simulink model "fftanalyzeri"  (R2012b)
settings: Solver=ode3  SolverMode=SingleTasking  StartTime=0.0  StopTime=20000  RelTol=1e-3
undefined symbols (not defined in the file or in its folder): pfb_coeff_gen_calc
undefined symbols (not defined in the file): fft_bin_flags_, magphmeanmem_, threshmem_
libraries: xbsIndex_r4 x9073, casper_library_misc x119, casper_library_flow_control x51, casper_library_delays x22, xps_library x10
(part 2 of 74)

== system fftanalyzeri/BinData ==
  addr : Inport
  data_in : Inport  Port=2
  we : Inport  Port=3
  calc_add : Subsystem  mask{data_width=32, addr_width=10, sample_rate=sample_rate}
      mask prompts: data_width "data width"; addr_width "address width"; sample_rate "sample rate"
  convert_addr : xbsIndex_r4/Convert  gui_display_data_type=Fixed-point  arith_type=Unsigned  n_bits=addr_width  bin_pt=0  float_type=Single  exp_bits=8  fraction_bits=24  quantization=Truncate  overflow=Wrap  en=off  latency=0  dbl_ovrd=off  pipeline=off  block_type=convert
      settings: xl_area=[0, 0, 0, 0, 0, 0, 0]
  convert_din1 : xbsIndex_r4/Convert  gui_display_data_type=Fixed-point  arith_type=Unsigned  n_bits=32  bin_pt=0  float_type=Single  exp_bits=8  fraction_bits=24  quantization=Truncate  overflow=Wrap  en=off  latency=0  dbl_ovrd=off  pipeline=off  block_type=convert
      settings: xl_area=[0, 0, 0, 0, 0, 0, 0]
  convert_we : xbsIndex_r4/Convert  gui_display_data_type=Fixed-point  arith_type=Unsigned  n_bits=1  bin_pt=0  float_type=Single  exp_bits=8  fraction_bits=24  quantization=Truncate  overflow=Wrap  en=off  latency=0  dbl_ovrd=off  pipeline=off  block_type=convert
      settings: xl_area=[0, 0, 0, 0, 0, 0, 0]
  fftanalyzeri_BinData_addr : xbsIndex_r4/Gateway Out  inherit_from_input=off  hdl_port=on  timing_constraint=None  locs_specified=off  LOCs={'A5','B9','A9','C1','A3','G6','E9','A6','A7','A8','B8','B1','B3','D9','B5','B4','B6','C2'}  UseAsDAC=off  DACChannel='1'  block_type=gatewayout
      settings: infoedit="Gateway out block.  Converts Xilinx fixed point inputs into ouputs of type Simulink integer, double, or fixed point.<P><P>Hardware notes:  In hardware these blocks become top level output ports or are discarded, depending on how they are configured."  xl_area=[0, 0, 0, 0, 0, 0, 0]  sginterface={'Nallatech'=>{'xdspkit'=>{'non_memory_mapped_port'=>'uprev_Shared_BRAM_addr'}},'Xilinx'=>{'jtaghwcosim'=>{'non_memory_mapped_port'=>'uprev_Shared_BRAM_addr'},'xdspkit'=>{'non_memory_mapped_port'=>'uprev_Shared_BRAM_addr'}}}
  fftanalyzeri_BinData_data_in : xbsIndex_r4/Gateway Out  inherit_from_input=off  hdl_port=on  timing_constraint=None  locs_specified=off  LOCs={'B21','B22','A22','B23','B19','C19','A20','A21','A23','B24','A24','A25','E18','D18','C18','B18'}  UseAsDAC=off  DACChannel='1'  block_type=gatewayout
      settings: infoedit="Gateway out block.  Converts Xilinx fixed point inputs into ouputs of type Simulink integer, double, or fixed point.<P><P>Hardware notes:  In hardware these blocks become top level output ports or are discarded, depending on how they are configured."  xl_area=[0, 0, 0, 0, 0, 0, 0]  sginterface={'Nallatech'=>{'xdspkit'=>{'non_memory_mapped_port'=>'uprev_Shared_BRAM_data_in'}},'Xilinx'=>{'jtaghwcosim'=>{'non_memory_mapped_port'=>'uprev_Shared_BRAM_data_in'},'xdspkit'=>{'non_memory_mapped_port'=>'uprev_Shared_BRAM_data_in'}}}
  fftanalyzeri_BinData_data_out : xbsIndex_r4/Gateway In  gui_display_data_type=Fixed-point  arith_type=Unsigned  n_bits=32  bin_pt=0  preci_type=Single  exp_width=8  frac_width=24  quantization=Truncate  overflow=Wrap  period=sample_rate  dbl_ovrd=off  timing_constraint=None  locs_specified=off  LOCs={}  UseAsADC=off  ADCChannel='1'  inherit_from_input=off  hdl_port=on  block_type=gatewayin
      settings: xl_area=[0, 0, 0, 0, 0, 0, 0]
  fftanalyzeri_BinData_we : xbsIndex_r4/Gateway Out  inherit_from_input=off  hdl_port=on  timing_constraint=None  locs_specified=off  LOCs={'A14'}  UseAsDAC=off  DACChannel='1'  block_type=gatewayout
      settings: infoedit="Gateway out block.  Converts Xilinx fixed point inputs into ouputs of type Simulink integer, double, or fixed point.<P><P>Hardware notes:  In hardware these blocks become top level output ports or are discarded, depending on how they are configured."  xl_area=[0, 0, 0, 0, 0, 0, 0]
  mem : Subsystem
  munge_in : Subsystem  AncestorBlock=casper_library_flow_control/munge  mask(munge){divisions=1, div_size=32, order=[0], arith_type_out=Unsigned, bin_pt_out=0}
      mask prompts: divisions "Number of divisions"; div_size "Division size (bits)"; order "Division packing order"; arith_type_out "Output arithmetic type"; bin_pt_out "Output binary point"
      mask help: Splits an input bus into the specified number of divisions and then recombines them in the order specified (most significant division = 0,least = number divisions-1)
      mask init:
      | munge_init(gcb, ...
      |     'divisions', divisions, ...
      |     'div_size', div_size, ...
      |     'order', order, ...
      |     'arith_type_out', arith_type_out, ...
      |     'bin_pt_out', bin_pt_out);
      settings: AttributesFormatString=|
      | split:32
      | join:0
      | Unsigned [32,0]
      mask TypeOptions arith_type_out: Unsigned | Signed  (2's comp) | Floating-point
  munge_out : Subsystem  AncestorBlock=casper_library_flow_control/munge  mask(munge){divisions=1, div_size=32, order=[0], arith_type_out=Unsigned, bin_pt_out=0}
      mask prompts: divisions "Number of divisions"; div_size "Division size (bits)"; order "Division packing order"; arith_type_out "Output arithmetic type"; bin_pt_out "Output binary point"
      mask help: Splits an input bus into the specified number of divisions and then recombines them in the order specified (most significant division = 0,least = number divisions-1)
      mask init:
      | munge_init(gcb, ...
      |     'divisions', divisions, ...
      |     'div_size', div_size, ...
      |     'order', order, ...
      |     'arith_type_out', arith_type_out, ...
      |     'bin_pt_out', bin_pt_out);
      settings: AttributesFormatString=|
      | split:32
      | join:0
      | Unsigned [32,0]
      mask TypeOptions arith_type_out: Unsigned | Signed  (2's comp) | Floating-point
  data_out : Outport
  wires:
  convert_addr/1 -> fftanalyzeri_BinData_addr/1
  convert_din1/1 -> fftanalyzeri_BinData_data_in/1
  data_in/1 -> munge_in/1(din)
  calc_add/1(out) -> convert_addr/1
  fftanalyzeri_BinData_we/1 -> mem/3(In3)
  fftanalyzeri_BinData_data_in/1 -> mem/2(In2)
  fftanalyzeri_BinData_addr/1 -> mem/1(In1)
  convert_we/1 -> fftanalyzeri_BinData_we/1
  fftanalyzeri_BinData_data_out/1 -> munge_out/1(din)
  mem/1(Out1) -> fftanalyzeri_BinData_data_out/1
  addr/1 -> calc_add/1(in)
  we/1 -> convert_we/1
  munge_out/1(dout) -> data_out/1
  munge_in/1(dout) -> convert_din1/1

== system fftanalyzeri/DRAM_LUT ==
  LUTsize : Inport
  startDAC : Inport  Port=2
  sys_sync : Inport  Port=3
  resetDRAM : Inport  Port=4
  RWen : Inport  Port=5
  holdcounter : Inport  Port=6
  seeaddress : Inport  Port=7
  Constant : xbsIndex_r4/Constant  const=0  gui_display_data_type=Fixed-point  arith_type=Unsigned  n_bits=32  bin_pt=0  preci_type=Single  exp_width=8  frac_width=24  explicit_period=off  period=1  equ=P=C  opselect=C  inp2=PCIN>>17  opr=+  inp1=P  carry=CIN  dbl_ovrd=off  block_type=constant
      settings: block_version=11.4
  Constant2 : xbsIndex_r4/Constant  const=0  gui_display_data_type=Fixed-point  arith_type=Unsigned  n_bits=144  bin_pt=0  preci_type=Single  exp_width=8  frac_width=24  explicit_period=on  period=1  equ=P=C  opselect=C  inp2=PCIN>>17  opr=+  inp1=P  carry=CIN  dbl_ovrd=off  block_type=constant
  Constant3 : xbsIndex_r4/Constant  const=0  gui_display_data_type=Fixed-point  arith_type=Unsigned  n_bits=36  bin_pt=0  preci_type=Single  exp_width=8  frac_width=24  explicit_period=on  period=1  equ=P=C  opselect=C  inp2=PCIN>>17  opr=+  inp1=P  carry=CIN  dbl_ovrd=off  block_type=constant
  Constant4 : xbsIndex_r4/Constant  const=0  gui_display_data_type=Fixed-point  arith_type=Unsigned  n_bits=32  bin_pt=0  preci_type=Single  exp_width=8  frac_width=24  explicit_period=on  period=1  equ=P=C  opselect=C  inp2=PCIN>>17  opr=+  inp1=P  carry=CIN  dbl_ovrd=off  block_type=constant
  Convert3 : xbsIndex_r4/Convert  gui_display_data_type=Fixed-point  arith_type=Unsigned  n_bits=32  bin_pt=0  float_type=Single  exp_bits=8  fraction_bits=24  quantization=Truncate  overflow=Wrap  en=off  latency=0  dbl_ovrd=off  pipeline=off  block_type=convert
      settings: block_version=10.1.3
  Counter1 : xbsIndex_r4/Counter  cnt_type=Free Running  cnt_to=511  operation=Up  start_count=0  cnt_by_val=1  arith_type=Unsigned  n_bits=32  bin_pt=0  load_pin=off  rst=on  en=on  explicit_period=on  period=1  dbl_ovrd=off  use_behavioral_HDL=off  implementation=Fabric  use_rpm=off  block_type=counter
  Counter2 : xbsIndex_r4/Counter  cnt_type=Free Running  cnt_to=512  operation=Up  start_count=0  cnt_by_val=1  arith_type=Unsigned  n_bits=32  bin_pt=0  load_pin=off  rst=on  en=on  explicit_period=on  period=1  dbl_ovrd=off  use_behavioral_HDL=off  implementation=Fabric  use_rpm=off  block_type=counter
  Delay4 : xbsIndex_r4/Delay  rst=off  infoeditControl=Selection of Reset will increase slice count due to use of real FFs and instead of SRLs  en=off  latency=2  dbl_ovrd=off  reg_retiming=off  block_type=delay
  Gateway Out{,1..7} (8 alike) : xbsIndex_r4/Gateway Out  inherit_from_input=off  hdl_port=on  timing_constraint=None  locs_specified=off  LOCs={}  UseAsDAC=off  DACChannel='1'  block_type=gatewayout
  Inverter1 : xbsIndex_r4/Inverter  en=off  latency=0  dbl_ovrd=off  block_type=inv
  Logical2 : xbsIndex_r4/Logical  logical_function=OR  inputs=2  en=off  latency=0  precision=Full  arith_type=Unsigned  n_bits=16  bin_pt=0  align_bp=on  dbl_ovrd=off  block_type=logical
  Mux : xbsIndex_r4/Mux  inputs=2  en=off  latency=0  precision=Full  arith_type=Unsigned  n_bits=16  bin_pt=14  quantization=Truncate  overflow=Wrap  dbl_ovrd=off  block_type=mux
      settings: block_version=11.4
  Mux1 : xbsIndex_r4/Mux  inputs=2  en=off  latency=0  precision=Full  arith_type=Unsigned  n_bits=16  bin_pt=14  quantization=Truncate  overflow=Wrap  dbl_ovrd=off  block_type=mux
  Reinterpret{1..8} (8 alike) : xbsIndex_r4/Reinterpret  force_arith_type=on  arith_type="Signed  (2's comp)"  force_bin_pt=on  bin_pt=15  block_type=reinterpret
      settings: infoedit="Changes signal type without altering the binary representation.   You can changed the signal between signed and unsigned, and relocate the binary point.<P><P>Hardware notes: In hardware this block costs nothing.<P><P>Example:  Suppose the input is 6 bits wide, signed, with 2 fractional bits, and the output is forced to unsigned with 0 fractional bits.  Then an input of -2.0 (1110.00 in binary 2's complement) becomes an output of 56 (111000 in binary)."  block_version=10.1.3
  Relational2 : xbsIndex_r4/Relational  mode=a=b  en=off  latency=0  dbl_ovrd=off  block_type=relational
      settings: block_version=10.1.3
  Slice10 : xbsIndex_r4/Slice  nbits=1  boolean_output=on  mode=Lower Bit Location + Width  bit1=0  base1=MSB of Input  bit0=0  base0=LSB of Input  dbl_ovrd=off  block_type=slice
      settings: infoedit="Extracts a given range of bits from each input sample and presents it at the output.  The output type is ordinarily unsigned with binary point at zero, but can be Boolean when the slice is one bit wide.<P><P>Hardware notes: In hardware this block costs nothing."  block_version=10.1.3
  Slice_16_0_ : xbsIndex_r4/Slice  nbits=16  boolean_output=off  mode=Lower Bit Location + Width  bit1=0  base1=LSB of Input  bit0=0  base0=LSB of Input  dbl_ovrd=off  block_type=slice
  Slice_16_0_1 : xbsIndex_r4/Slice  nbits=16  boolean_output=off  mode=Lower Bit Location + Width  bit1=0  base1=LSB of Input  bit0=0  base0=LSB of Input  dbl_ovrd=off  block_type=slice
  Slice_16_104_6 : xbsIndex_r4/Slice  nbits=16  boolean_output=off  mode=Lower Bit Location + Width  bit1=0  base1=LSB of Input  bit0=104  base0=LSB of Input  dbl_ovrd=off  block_type=slice
  Slice_16_120_7 : xbsIndex_r4/Slice  nbits=16  boolean_output=off  mode=Lower Bit Location + Width  bit1=0  base1=LSB of Input  bit0=120  base0=LSB of Input  dbl_ovrd=off  block_type=slice
  Slice_16_16_1 : xbsIndex_r4/Slice  nbits=16  boolean_output=off  mode=Lower Bit Location + Width  bit1=0  base1=LSB of Input  bit0=16  base0=LSB of Input  dbl_ovrd=off  block_type=slice
  Slice_16_32_2 : xbsIndex_r4/Slice  nbits=16  boolean_output=off  mode=Lower Bit Location + Width  bit1=0  base1=LSB of Input  bit0=32  base0=LSB of Input  dbl_ovrd=off  block_type=slice
  Slice_16_64_3 : xbsIndex_r4/Slice  nbits=16  boolean_output=off  mode=Lower Bit Location + Width  bit1=0  base1=LSB of Input  bit0=48  base0=LSB of Input  dbl_ovrd=off  block_type=slice
  Slice_16_72_4 : xbsIndex_r4/Slice  nbits=16  boolean_output=off  mode=Lower Bit Location + Width  bit1=0  base1=LSB of Input  bit0=72  base0=LSB of Input  dbl_ovrd=off  block_type=slice
  Slice_16_88_5 : xbsIndex_r4/Slice  nbits=16  boolean_output=off  mode=Lower Bit Location + Width  bit1=0  base1=LSB of Input  bit0=88  base0=LSB of Input  dbl_ovrd=off  block_type=slice
  dram : xps_library/dram  Tag=xps:dram  dimm=1  arith_type=Unsigned  bin_pt=0  ip_clock=200  sample_period=1  bram_fifos=on  disable_tag=off  ram_depth=18  bank_mgt=off  wide_data=off  half_burst=off  use_sniffer=on
  memscope : Scope  NumInputPorts=8
      settings: YMin=-5~-5~-5~-5~-5~-5~-5~-5  YMax=5~5~5~5~5~5~5~5
  posedge : casper_library_misc/posedge  Tag=Rising Edge Detector
  posedge2 : casper_library_misc/posedge  Tag=Rising Edge Detector
  data_i0 : Outport
  data_i1 : Outport  Port=2
  data_i2 : Outport  Port=3
  data_i3 : Outport  Port=4
  data_q0 : Outport  Port=5
  data_q1 : Outport  Port=6
  data_q2 : Outport  Port=7
  data_q3 : Outport  Port=8
  sync_out : Outport  Port=9
  wires:
  resetDRAM/1 -> dram/1, Gateway Out/1
  RWen/1 -> Gateway Out2/1, dram/5, dram/8
  Constant2/1 -> dram/3
  Constant3/1 -> dram/4
  Counter2/1 -> Relational2/2, Gateway Out4/1, Mux/2
  Counter1/1 -> Slice10/1
  Slice10/1 -> posedge2/1
  Convert3/1 -> Relational2/1
  posedge2/1 -> Counter2/2, Delay4/1
  Constant4/1 -> dram/6
  Delay4/1 -> Gateway Out3/1, dram/7
  LUTsize/1 -> Convert3/1
  Slice_16_16_1/1 -> Reinterpret1/1
  Slice_16_104_6/1 -> Reinterpret3/1
  Slice_16_120_7/1 -> Reinterpret2/1
  Slice_16_32_2/1 -> Reinterpret5/1
  Slice_16_64_3/1 -> Reinterpret6/1
  Slice_16_88_5/1 -> Reinterpret7/1
  Slice_16_72_4/1 -> Reinterpret8/1
  Reinterpret4/1 -> data_i0/1
  Reinterpret1/1 -> data_i1/1
  Reinterpret5/1 -> data_i2/1
  Reinterpret6/1 -> data_i3/1
  Reinterpret8/1 -> data_q0/1
  Reinterpret7/1 -> data_q1/1
  Reinterpret3/1 -> data_q2/1
  Reinterpret2/1 -> data_q3/1
  startDAC/1 -> Inverter1/1, Counter1/2
  Logical2/1 -> Counter2/1
  Relational2/1 -> posedge/1, Logical2/1
  Inverter1/1 -> Logical2/2
  sys_sync/1 -> Counter1/1
  Mux/1 -> dram/2, Slice_16_0_1/1, Gateway Out1/1
  Constant/1 -> Mux/3
  holdcounter/1 -> Mux/1
  Gateway Out/1 -> memscope/1
  Gateway Out1/1 -> memscope/2
  Gateway Out2/1 -> memscope/3
  Gateway Out3/1 -> memscope/4
  Gateway Out4/1 -> memscope/5
  Gateway Out5/1 -> memscope/6
  dram/2 -> Slice_16_120_7/1, Slice_16_104_6/1, Slice_16_88_5/1, Slice_16_72_4/1, Slice_16_64_3/1, Slice_16_32_2/1, Slice_16_16_1/1, Slice_16_0_/1, Gateway Out7/1
  Gateway Out7/1 -> memscope/7
  Gateway Out6/1 -> memscope/8
  dram/4 -> Gateway Out6/1
  dram/1 -> Gateway Out5/1
  Slice_16_0_/1 -> Mux1/2
  Mux1/1 -> Reinterpret4/1
  Slice_16_0_1/1 -> Mux1/3
  seeaddress/1 -> Mux1/1
  posedge/1 -> sync_out/1

== system fftanalyzeri/FIFO64_ ==
  chanwr : Inport
  wr : Inport  Port=2
  din : Inport  Port=3
  chanrd : Inport  Port=4
  rd : Inport  Port=5
  rst : Inport  Port=6
  rden : Inport  Port=7
  wren : Inport  Port=8
  FIFO32_0 : Subsystem
  FIFO32_1 : Subsystem
  Gateway Out{1..16} (16 alike) : xbsIndex_r4/Gateway Out  inherit_from_input=off  hdl_port=on  timing_constraint=None  locs_specified=off  LOCs={}  UseAsDAC=off  DACChannel='1'  block_type=gatewayout
  Subsystem1 : Subsystem
  Subsystem2 : Subsystem
  fifoscope1 : Scope  NumInputPorts=8
      settings: YMin=-5~-5~-5~-5~-5~-5~-5~-5  YMax=5~5~5~5~5~5~5~5  SaveName=fsmdata6
  fifoscope2 : Scope  NumInputPorts=8
      settings: YMin=-5~-5~-5~-5~-5~-5~-5~-5  YMax=5~5~5~5~5~5~5~5  SaveName=fsmdata7
  q : Outport
  empty : Outport  Port=2
  halffull : Outport  Port=3
  quartfull : Outport  Port=4
  threeqfull : Outport  Port=5
  full : Outport  Port=6
  fifllen : Outport  Port=7
  dvld : Outport  Port=8
  wires:
  wr/1 -> Gateway Out10/1, FIFO32_1/2(wr), FIFO32_0/2(wr)
  rst/1 -> FIFO32_1/6(rst), FIFO32_0/6(rst)
  chanrd/1 -> Gateway Out9/1, Subsystem2/2(chanrd), Subsystem1/4(In4), FIFO32_1/4(chanrd), FIFO32_0/4(chanrd)
  din/1 -> FIFO32_1/3(din), FIFO32_0/3(din)
  chanwr/1 -> Gateway Out8/1, Subsystem2/1(chanwr), FIFO32_1/1(chanwr), FIFO32_0/1(chanwr)
  rd/1 -> Gateway Out11/1, FIFO32_1/5(rd), FIFO32_0/5(rd)
  FIFO32_0/1(q) -> Subsystem1/1(In1)
  FIFO32_0/2(empty) -> Gateway Out7/1, Subsystem1/2(In2)
  FIFO32_0/3(halffull) -> Gateway Out1/1, Subsystem1/3(In3)
  FIFO32_0/4(quartfull) -> Gateway Out2/1, Subsystem1/5(In5)
  FIFO32_0/5(threeqfull) -> Subsystem1/6(In6)
  FIFO32_0/6(full) -> Subsystem1/7(In7)
  FIFO32_0/7(fifllen) -> Gateway Out16/1, Subsystem1/8(In8)
  FIFO32_0/8(dvld) -> Subsystem1/9(In9)
  FIFO32_1/1(q) -> Subsystem1/10(In10)
  FIFO32_1/2(empty) -> Gateway Out3/1, Subsystem1/11(In11)
  FIFO32_1/3(halffull) -> Subsystem1/12(In12)
  FIFO32_1/4(quartfull) -> Gateway Out5/1, Subsystem1/13(In13)
  FIFO32_1/5(threeqfull) -> Gateway Out6/1, Subsystem1/14(In14)
  FIFO32_1/6(full) -> Subsystem1/15(In15)
  FIFO32_1/7(fifllen) -> Gateway Out4/1, Subsystem1/16(In16)
  FIFO32_1/8(dvld) -> Subsystem1/17(In17)
  Subsystem1/1(Out1) -> q/1
  Subsystem1/2(Out2) -> empty/1
  Subsystem1/3(Out3) -> halffull/1
  Subsystem1/4(Out4) -> quartfull/1
  Subsystem1/5(Out5) -> threeqfull/1
  Subsystem1/6(Out6) -> full/1
  Subsystem1/7(Out7) -> fifllen/1
  Subsystem1/8(Out8) -> dvld/1
  rden/1 -> Subsystem2/3(rden)
  wren/1 -> Subsystem2/4(wren)
  Subsystem2/2(rdl) -> Gateway Out13/1, FIFO32_0/7(rden)
  Subsystem2/3(wrh) -> Gateway Out14/1, FIFO32_1/8(wren)
  Subsystem2/1(wrl) -> Gateway Out12/1, FIFO32_0/8(wren)
  Subsystem2/4(rdh) -> Gateway Out15/1, FIFO32_1/7(rden)
  Gateway Out8/1 -> fifoscope1/1
  Gateway Out9/1 -> fifoscope1/2
  Gateway Out10/1 -> fifoscope1/3
  Gateway Out11/1 -> fifoscope1/4
  Gateway Out12/1 -> fifoscope1/5
  Gateway Out13/1 -> fifoscope1/6
  Gateway Out14/1 -> fifoscope1/7
  Gateway Out15/1 -> fifoscope1/8
  Gateway Out7/1 -> fifoscope2/1
  Gateway Out16/1 -> fifoscope2/2
  Gateway Out1/1 -> fifoscope2/3
  Gateway Out2/1 -> fifoscope2/4
  Gateway Out3/1 -> fifoscope2/5
  Gateway Out4/1 -> fifoscope2/6
  Gateway Out5/1 -> fifoscope2/7
  Gateway Out6/1 -> fifoscope2/8

== system fftanalyzeri/FIFO64_1 ==
  chanwr : Inport
  wr : Inport  Port=2
  din : Inport  Port=3
  chanrd : Inport  Port=4
  rd : Inport  Port=5
  rst : Inport  Port=6
  rden : Inport  Port=7
  wren : Inport  Port=8
  FIFO32_0 : Subsystem
  FIFO32_1 : Subsystem
  Subsystem1 : Subsystem
  Subsystem2 : Subsystem
  q : Outport
  empty : Outport  Port=2
  halffull : Outport  Port=3
  quartfull : Outport  Port=4
  threeqfull : Outport  Port=5
  full : Outport  Port=6
  fifllen : Outport  Port=7
  dvld : Outport  Port=8
  wires:
  wr/1 -> FIFO32_1/2(wr), FIFO32_0/2(wr)
  rst/1 -> FIFO32_1/6(rst), FIFO32_0/6(rst)
  chanrd/1 -> Subsystem2/2(chanrd), Subsystem1/4(In4), FIFO32_1/4(chanrd), FIFO32_0/4(chanrd)
  din/1 -> FIFO32_1/3(din), FIFO32_0/3(din)
  chanwr/1 -> Subsystem2/1(chanwr), FIFO32_1/1(chanwr), FIFO32_0/1(chanwr)
  rd/1 -> FIFO32_1/5(rd), FIFO32_0/5(rd)
  FIFO32_0/1(q) -> Subsystem1/1(In1)
  FIFO32_0/2(empty) -> Subsystem1/2(In2)
  FIFO32_0/3(halffull) -> Subsystem1/3(In3)
  FIFO32_0/4(quartfull) -> Subsystem1/5(In5)
  FIFO32_0/5(threeqfull) -> Subsystem1/6(In6)
  FIFO32_0/6(full) -> Subsystem1/7(In7)
  FIFO32_0/7(fifllen) -> Subsystem1/8(In8)
  FIFO32_0/8(dvld) -> Subsystem1/9(In9)
  FIFO32_1/1(q) -> Subsystem1/10(In10)
  FIFO32_1/2(empty) -> Subsystem1/11(In11)
  FIFO32_1/3(halffull) -> Subsystem1/12(In12)
  FIFO32_1/4(quartfull) -> Subsystem1/13(In13)
  FIFO32_1/5(threeqfull) -> Subsystem1/14(In14)
  FIFO32_1/6(full) -> Subsystem1/15(In15)
  FIFO32_1/7(fifllen) -> Subsystem1/16(In16)
  FIFO32_1/8(dvld) -> Subsystem1/17(In17)
  Subsystem1/1(Out1) -> q/1
  Subsystem1/2(Out2) -> empty/1
  Subsystem1/3(Out3) -> halffull/1
  Subsystem1/4(Out4) -> quartfull/1
  Subsystem1/5(Out5) -> threeqfull/1
  Subsystem1/6(Out6) -> full/1
  Subsystem1/7(Out7) -> fifllen/1
  Subsystem1/8(Out8) -> dvld/1
  rden/1 -> Subsystem2/3(rden)
  wren/1 -> Subsystem2/4(wren)
  Subsystem2/2(rdl) -> FIFO32_0/7(rden)
  Subsystem2/3(wrh) -> FIFO32_1/8(wren)
  Subsystem2/1(wrl) -> FIFO32_0/8(wren)
  Subsystem2/4(rdh) -> FIFO32_1/7(rden)

== system fftanalyzeri/FIFO64_2 ==
  chanwr : Inport
  wr : Inport  Port=2
  din : Inport  Port=3
  chanrd : Inport  Port=4
  rd : Inport  Port=5
  rst : Inport  Port=6
  rden : Inport  Port=7
  wren : Inport  Port=8
  FIFO32_0 : Subsystem
  FIFO32_1 : Subsystem
  Subsystem1 : Subsystem
  Subsystem2 : Subsystem
  q : Outport
  empty : Outport  Port=2
  halffull : Outport  Port=3
  quartfull : Outport  Port=4
  threeqfull : Outport  Port=5
  full : Outport  Port=6
  fifllen : Outport  Port=7
  dvld : Outport  Port=8
  wires:
  wr/1 -> FIFO32_1/2(wr), FIFO32_0/2(wr)
  rst/1 -> FIFO32_1/6(rst), FIFO32_0/6(rst)
  chanrd/1 -> Subsystem2/2(chanrd), Subsystem1/4(In4), FIFO32_1/4(chanrd), FIFO32_0/4(chanrd)
  din/1 -> FIFO32_1/3(din), FIFO32_0/3(din)
  chanwr/1 -> Subsystem2/1(chanwr), FIFO32_1/1(chanwr), FIFO32_0/1(chanwr)
  rd/1 -> FIFO32_1/5(rd), FIFO32_0/5(rd)
  FIFO32_0/1(q) -> Subsystem1/1(In1)
  FIFO32_0/2(empty) -> Subsystem1/2(In2)
  FIFO32_0/3(halffull) -> Subsystem1/3(In3)
  FIFO32_0/4(quartfull) -> Subsystem1/5(In5)
  FIFO32_0/5(threeqfull) -> Subsystem1/6(In6)
  FIFO32_0/6(full) -> Subsystem1/7(In7)
  FIFO32_0/7(fifllen) -> Subsystem1/8(In8)
  FIFO32_0/8(dvld) -> Subsystem1/9(In9)
  FIFO32_1/1(q) -> Subsystem1/10(In10)
  FIFO32_1/2(empty) -> Subsystem1/11(In11)
  FIFO32_1/3(halffull) -> Subsystem1/12(In12)
  FIFO32_1/4(quartfull) -> Subsystem1/13(In13)
  FIFO32_1/5(threeqfull) -> Subsystem1/14(In14)
  FIFO32_1/6(full) -> Subsystem1/15(In15)
  FIFO32_1/7(fifllen) -> Subsystem1/16(In16)
  FIFO32_1/8(dvld) -> Subsystem1/17(In17)
  Subsystem1/1(Out1) -> q/1
  Subsystem1/2(Out2) -> empty/1
  Subsystem1/3(Out3) -> halffull/1
  Subsystem1/4(Out4) -> quartfull/1
  Subsystem1/5(Out5) -> threeqfull/1
  Subsystem1/6(Out6) -> full/1
  Subsystem1/7(Out7) -> fifllen/1
  Subsystem1/8(Out8) -> dvld/1
  rden/1 -> Subsystem2/3(rden)
  wren/1 -> Subsystem2/4(wren)
  Subsystem2/2(rdl) -> FIFO32_0/7(rden)
  Subsystem2/3(wrh) -> FIFO32_1/8(wren)
  Subsystem2/1(wrl) -> FIFO32_0/8(wren)
  Subsystem2/4(rdh) -> FIFO32_1/7(rden)

== system fftanalyzeri/FIFO64_3 ==
  chanwr : Inport
  wr : Inport  Port=2
  din : Inport  Port=3
  chanrd : Inport  Port=4
  rd : Inport  Port=5
  rst : Inport  Port=6
  rden : Inport  Port=7
  wren : Inport  Port=8
  FIFO32_0 : Subsystem
  FIFO32_1 : Subsystem
  Subsystem1 : Subsystem
  Subsystem2 : Subsystem
  q : Outport
  empty : Outport  Port=2
  halffull : Outport  Port=3
  quartfull : Outport  Port=4
  threeqfull : Outport  Port=5
  full : Outport  Port=6
  fifllen : Outport  Port=7
  dvld : Outport  Port=8
  wires:
  wr/1 -> FIFO32_1/2(wr), FIFO32_0/2(wr)
  rst/1 -> FIFO32_1/6(rst), FIFO32_0/6(rst)
  chanrd/1 -> Subsystem2/2(chanrd), Subsystem1/4(In4), FIFO32_1/4(chanrd), FIFO32_0/4(chanrd)
  din/1 -> FIFO32_1/3(din), FIFO32_0/3(din)
  chanwr/1 -> Subsystem2/1(chanwr), FIFO32_1/1(chanwr), FIFO32_0/1(chanwr)
  rd/1 -> FIFO32_1/5(rd), FIFO32_0/5(rd)
  FIFO32_0/1(q) -> Subsystem1/1(In1)
  FIFO32_0/2(empty) -> Subsystem1/2(In2)
  FIFO32_0/3(halffull) -> Subsystem1/3(In3)
  FIFO32_0/4(quartfull) -> Subsystem1/5(In5)
  FIFO32_0/5(threeqfull) -> Subsystem1/6(In6)
  FIFO32_0/6(full) -> Subsystem1/7(In7)
  FIFO32_0/7(fifllen) -> Subsystem1/8(In8)
  FIFO32_0/8(dvld) -> Subsystem1/9(In9)
  FIFO32_1/1(q) -> Subsystem1/10(In10)
  FIFO32_1/2(empty) -> Subsystem1/11(In11)
  FIFO32_1/3(halffull) -> Subsystem1/12(In12)
  FIFO32_1/4(quartfull) -> Subsystem1/13(In13)
  FIFO32_1/5(threeqfull) -> Subsystem1/14(In14)
  FIFO32_1/6(full) -> Subsystem1/15(In15)
  FIFO32_1/7(fifllen) -> Subsystem1/16(In16)
  FIFO32_1/8(dvld) -> Subsystem1/17(In17)
  Subsystem1/1(Out1) -> q/1
  Subsystem1/2(Out2) -> empty/1
  Subsystem1/3(Out3) -> halffull/1
  Subsystem1/4(Out4) -> quartfull/1
  Subsystem1/5(Out5) -> threeqfull/1
  Subsystem1/6(Out6) -> full/1
  Subsystem1/7(Out7) -> fifllen/1
  Subsystem1/8(Out8) -> dvld/1
  rden/1 -> Subsystem2/3(rden)
  wren/1 -> Subsystem2/4(wren)
  Subsystem2/2(rdl) -> FIFO32_0/7(rden)
  Subsystem2/3(wrh) -> FIFO32_1/8(wren)
  Subsystem2/1(wrl) -> FIFO32_0/8(wren)
  Subsystem2/4(rdh) -> FIFO32_1/7(rden)

== system fftanalyzeri/LO_SLE ==
  sim_reg : Inport
  fftanalyzeri_LO_SLE_user_data_out : xbsIndex_r4/Gateway In  gui_display_data_type=Fixed-point  arith_type=Unsigned  n_bits=32  bin_pt=0  preci_type=Single  exp_width=8  frac_width=24  quantization="Round  (unbiased: +/- Inf)"  overflow=Saturate  period=1  dbl_ovrd=off  timing_constraint=None  locs_specified=off  LOCs={}  UseAsADC=off  ADCChannel='1'  inherit_from_input=off  hdl_port=on  block_type=gatewayin
  io_delay : xbsIndex_r4/Delay  rst=off  infoeditControl=Selection of Reset will increase slice count due to use of real FFs and instead of SRLs  en=off  latency=0  dbl_ovrd=off  reg_retiming=on  block_type=delay
  reint1 : xbsIndex_r4/Reinterpret  force_arith_type=on  arith_type=Unsigned  force_bin_pt=on  bin_pt=0  block_type=reinterpret
  slice_reg : xbsIndex_r4/Slice  nbits=32  boolean_output=off  mode=Lower Bit Location + Width  bit1=0  base1=MSB of Input  bit0=0  base0=LSB of Input  dbl_ovrd=off  block_type=slice
  in_reg : Outport
  wires:
  fftanalyzeri_LO_SLE_user_data_out/1 -> io_delay/1
  sim_reg/1 -> fftanalyzeri_LO_SLE_user_data_out/1
  io_delay/1 -> slice_reg/1
  slice_reg/1 -> reint1/1
  reint1/1 -> in_reg/1

== system fftanalyzeri/LUTsize ==
  sim_reg : Inport
  fftanalyzeri_LUTsize_user_data_out : xbsIndex_r4/Gateway In  gui_display_data_type=Fixed-point  arith_type=Unsigned  n_bits=32  bin_pt=0  preci_type=Single  exp_width=8  frac_width=24  quantization="Round  (unbiased: +/- Inf)"  overflow=Saturate  period=1  dbl_ovrd=off  timing_constraint=None  locs_specified=off  LOCs={}  UseAsADC=off  ADCChannel='1'  inherit_from_input=off  hdl_port=on  block_type=gatewayin
  io_delay : xbsIndex_r4/Delay  rst=off  infoeditControl=Selection of Reset will increase slice count due to use of real FFs and instead of SRLs  en=off  latency=0  dbl_ovrd=off  reg_retiming=on  block_type=delay
  reint1 : xbsIndex_r4/Reinterpret  force_arith_type=on  arith_type=Unsigned  force_bin_pt=on  bin_pt=0  block_type=reinterpret
  slice_reg : xbsIndex_r4/Slice  nbits=32  boolean_output=off  mode=Lower Bit Location + Width  bit1=0  base1=MSB of Input  bit0=0  base0=LSB of Input  dbl_ovrd=off  block_type=slice
  in_reg : Outport
  wires:
  fftanalyzeri_LUTsize_user_data_out/1 -> io_delay/1
  sim_reg/1 -> fftanalyzeri_LUTsize_user_data_out/1
  io_delay/1 -> slice_reg/1
  slice_reg/1 -> reint1/1
  reint1/1 -> in_reg/1

== system fftanalyzeri/MemRecordPolar ==
  note: 17 bits
  note: Size is set by this:
      | set const 6, and width of const 6
      | Set width of counter
      | Set depth of BRAM
  Start : Inport
  DataIn : Inport  Port=2
  WE : Inport  Port=3
  Delay1 : xbsIndex_r4/Delay  rst=off  infoeditControl=Selection of Reset will increase slice count due to use of real FFs and instead of SRLs  en=off  latency=1  dbl_ovrd=off  reg_retiming=off  block_type=delay
  Delay2 : xbsIndex_r4/Delay  rst=off  infoeditControl=Selection of Reset will increase slice count due to use of real FFs and instead of SRLs  en=off  latency=1  dbl_ovrd=off  reg_retiming=off  block_type=delay
  Delay3 : xbsIndex_r4/Delay  rst=off  infoeditControl=Selection of Reset will increase slice count due to use of real FFs and instead of SRLs  en=off  latency=1  dbl_ovrd=off  reg_retiming=off  block_type=delay
  Gateway Out{1..8} (8 alike) : xbsIndex_r4/Gateway Out  inherit_from_input=off  hdl_port=off  timing_constraint=None  locs_specified=off  LOCs={}  UseAsDAC=off  DACChannel='1'  block_type=gatewayout
  Inverter : xbsIndex_r4/Inverter  en=off  latency=0  dbl_ovrd=off  block_type=inv
  Logical : xbsIndex_r4/Logical  logical_function=AND  inputs=2  en=off  latency=0  precision=Full  arith_type=Unsigned  n_bits=16  bin_pt=0  align_bp=on  dbl_ovrd=off  block_type=logical
  Relational : xbsIndex_r4/Relational  mode=a=b  en=off  latency=0  dbl_ovrd=off  block_type=relational
  Shared BRAM : Subsystem  Tag=xps:bram  AncestorBlock=xps_library/Shared BRAM  mask{arith_type=Unsigned, addr_width=15, data_width=32, reg_prim_output=off, reg_core_output=off, optimization=Minimum_Area, data_bin_pt=0, init_vals=[0:2^10-1], sample_rate=1}
      mask prompts: arith_type "Output Data Type"; addr_width "Address width"; data_width "Data Width"; reg_prim_output "Register Primitive Output"; reg_core_output "Register Core Output"; data_bin_pt "Data Binary Point"; init_vals "Initial values (simulation only)"; sample_rate "Sample rate"
      mask init:
      | shared_bram_mask;
      mask TypeOptions arith_type: Unsigned | Signed  (2's comp)
      mask TypeOptions data_width: 8 | 16 | 32 | 64 | 128
      mask TypeOptions optimization: Minimum_Area | Low_Power
  Terminator1 : Terminator
  Terminator13 : Terminator
  bits0_15_ : xbsIndex_r4/Slice  nbits=15  boolean_output=off  mode=Lower Bit Location + Width  bit1=0  base1=MSB of Input  bit0=0  base0=LSB of Input  dbl_ovrd=off  block_type=slice
  coefRamAddr : Subsystem  Tag=xps:sw_reg  AncestorBlock=xps_library/software register  mask{numios=1, io_dir=To Processor, io_delay=0, sample_period=1, name1=reg, bitwidth1=32, arith_type1=Unsigned, bin_pt1=0}
      mask prompts: numios "Num I/Os"; io_dir "I/O direction"; io_delay "I/O delay"; sample_period "Sample period"; name1 "Name"; bitwidth1 "Bitwidth"; arith_type1 "Type"; bin_pt1 "Binary pt"
      mask init:
      | swreg_init(gcb);
      mask Callback numios: t = timer('StartDelay', 0.1); t.TimerFcn = {@swreg_cb, gcb}; start(t);
      mask TypeOptions io_dir: To Processor | From Processor
      mask Callback io_dir:
      | a = get_param(gcb, 'MaskEnables');
      | if strcmp(get_param(gcb, 'io_dir'), 'To Processor'),
      | a(4) = {'off'};
      | else
      | a(4) = {'on'};
      | end
      | set_param(gcb, 'MaskEnables', a);
      mask TypeOptions arith_type1: Unsigned | Signed  (2's comp) | Boolean
      mask Callback arith_type1:
      | a = get_param(gcb, 'MaskEnables');
      | if strcmp(get_param(gcb, 'arith_type1'), 'Boolean'),
      | set_param(gcb, 'bitwidth1', '1');
      | set_param(gcb, 'bin_pt1', '0');
      | a(6) = {'off'};
      | a(8) = {'off'};
      | else
      | a(6) = {'on'};
      | a(8) = {'on'};
      | end
      | set_param(gcb, 'MaskEnables', a);
  const17bit_ : xbsIndex_r4/Constant  const=32768  gui_display_data_type=Fixed-point  arith_type=Unsigned  n_bits=17  bin_pt=0  preci_type=Single  exp_width=8  frac_width=24  explicit_period=on  period=1  equ=P=C  opselect=C  inp2=PCIN>>17  opr=+  inp1=P  carry=CIN  dbl_ovrd=off  block_type=constant
  edge_detect : casper_library_misc/edge_detect  edge=Rising  polarity=Active High  x_in=[0 0.08 0.08 0.16 0.16 0.24 0.24 0.32 0.32 0.4]  y_in="[-1 -1  1  1  1  1  1  1  1  1]"  x_out=[0.6 0.68 0.68 0.76 0.76 0.84 0.84 0.92 0.92 1]  y_out="[-1 -1  1  1 -1 -1 -1 -1 -1 -1]"
  memrecordscope : Scope  NumInputPorts=8
      settings: YMin=0~-5~-5~-5~-5~-5~-5~-5  YMax=300000~5~5~5~5~5~5~5  MaxDataPoints=10000
  spect_cnt : xbsIndex_r4/Counter  cnt_type=Free Running  cnt_to=Inf  operation=Up  start_count=0  cnt_by_val=1  arith_type=Unsigned  n_bits=17  bin_pt=0  load_pin=off  rst=on  en=on  explicit_period=on  period=1  dbl_ovrd=off  use_behavioral_HDL=off  implementation=Fabric  use_rpm=off  block_type=counter
  memDone : Outport
  wires:
  spect_cnt/1 -> bits0_15_/1, Relational/2, coefRamAddr/1(out_reg), Gateway Out2/1
  const17bit_/1 -> Relational/1
  WE/1 -> Logical/2, Gateway Out6/1
  Gateway Out5/1 -> memrecordscope/1
  Gateway Out1/1 -> memrecordscope/2
  Gateway Out2/1 -> memrecordscope/3
  Gateway Out3/1 -> memrecordscope/4
  Gateway Out4/1 -> memrecordscope/5
  Gateway Out6/1 -> memrecordscope/6
  Delay1/1 -> Shared BRAM/1(addr)
  Delay3/1 -> Shared BRAM/2(data_in)
  Delay2/1 -> Shared BRAM/3(we)
  Gateway Out7/1 -> memrecordscope/7
  Gateway Out8/1 -> memrecordscope/8
  coefRamAddr/1(sim_out) -> Terminator1/1
  bits0_15_/1 -> Delay1/1
  Logical/1 -> spect_cnt/2, Gateway Out7/1, Delay2/1
  Shared BRAM/1(data_out) -> Terminator13/1
  Relational/1 -> Inverter/1, Gateway Out3/1, memDone/1
  Inverter/1 -> Gateway Out4/1, Logical/1
  DataIn/1 -> Gateway Out8/1, Delay3/1
  edge_detect/1 -> Gateway Out1/1, spect_cnt/1
  Start/1 -> Gateway Out5/1, edge_detect/1

== system fftanalyzeri/PhaseCorrect1 ==
  note: 1 for prog mode, 0 for run mode
  note: WE for prog phase inc
  note: Registers to clear phase accum and prog phase incs
      | from linux
  note: phase increment per sample
      | we can prog them from linux
  note: array of counters.
      | we can clear them from l;inmux
  note: inc amount
  note: chan prog
  note: prog or run
  note: Clear accum at addr
  note: Phase comes in as 18,15. That means we can represent from -4pi to +4pi. Dont know why are doing this. it should be 0 to 2pi and that is all.
      | The cordic alg outputs phase from -pi to +pi. so we want to take the simmed data and force it into -pi to +pi.
      | We can reintrepret the lower 16 bits as i16.15.
  note: it is still in polar cord.
  note: Assume that data is mag, phase.
      | phase is im part
  note: Present chan, data in, and dvld in at same clock
      | You can present chan any abount of clocks early as well.
      | when chaning chan, need to incl extra pipeline, or clock, to make sure data is written correctl.
      | best operation:
      | 1 sett chan
      | 2 set data, and dvld, for many clocks, however long data is
      | 3 turn off dvls
      |  4  goto 1
  note: Add phase to the incommign data.
      | this takes out const. rotation of fft coef data
      | when source sin is not at bin center.
      | Because each channel has unique phase offset,
  note: per channel basis
  note: Bank of phase increments
      | per channel basis
  note: Bank of phase accums.
  dvld_in : Inport
  cmplx_din : Inport  Port=2
  chan : Inport  Port=3
  en : Inport  Port=4
  clrPhase : Inport  Port=5
  AddSub1 : xbsIndex_r4/AddSub  mode=Addition  use_carryin=off  use_carryout=off  en=on  latency=1  precision=User Defined  arith_type="Signed  (2's comp)"  n_bits=16  bin_pt=15  quantization=Truncate  overflow=Wrap  dbl_ovrd=off  use_behavioral_HDL=off  hw_selection=Fabric  pipelined=off  block_type=addsub
  AddSub2 : xbsIndex_r4/AddSub  mode=Addition  use_carryin=off  use_carryout=off  en=off  latency=0  precision=User Defined  arith_type="Signed  (2's comp)"  n_bits=32  bin_pt=30  quantization=Truncate  overflow=Wrap  dbl_ovrd=off  use_behavioral_HDL=off  hw_selection=Fabric  pipelined=off  block_type=addsub
  Constant : xbsIndex_r4/Constant  const=256  gui_display_data_type=Fixed-point  arith_type=Unsigned  n_bits=9  bin_pt=0  preci_type=Single  exp_width=8  frac_width=24  explicit_period=on  period=1  equ=P=C  opselect=C  inp2=PCIN>>17  opr=+  inp1=P  carry=CIN  dbl_ovrd=off  block_type=constant
  Counter : xbsIndex_r4/Counter  cnt_type=Free Running  cnt_to=Inf  operation=Up  start_count=0  cnt_by_val=1  arith_type=Unsigned  n_bits=9  bin_pt=0  load_pin=off  rst=on  en=on  explicit_period=on  period=1  dbl_ovrd=off  use_behavioral_HDL=off  implementation=Fabric  block_type=counter
  Delay : xbsIndex_r4/Delay  rst=off  infoeditControl=Selection of Reset will increase slice count due to use of real FFs and instead of SRLs  en=on  latency=2  dbl_ovrd=off  reg_retiming=off  block_type=delay
  Delay1 : xbsIndex_r4/Delay  rst=off  infoeditControl=Selection of Reset will increase slice count due to use of real FFs and instead of SRLs  en=on  latency=1  dbl_ovrd=off  reg_retiming=off  block_type=delay
  Delay2 : xbsIndex_r4/Delay  rst=off  infoeditControl=Selection of Reset will increase slice count due to use of real FFs and instead of SRLs  en=on  latency=2  dbl_ovrd=off  reg_retiming=off  block_type=delay
  Delay3 : xbsIndex_r4/Delay  rst=off  infoeditControl=Selection of Reset will increase slice count due to use of real FFs and instead of SRLs  en=on  latency=1  dbl_ovrd=off  reg_retiming=off  block_type=delay
  From Workspace : FromWorkspace  VariableName=PhaseCorrect1_phaseIncVal  SampleTime=0  OutputAfterFinalValue=Holding final value
  From Workspace1 : FromWorkspace  VariableName=PhaseCorrect1_phaseIncAddr  SampleTime=0
  From Workspace2 : FromWorkspace  VariableName=PhaseCorrect1_phaseIncProgWe  SampleTime=0
  Gateway Out{,1..7} (8 alike) : xbsIndex_r4/Gateway Out  inherit_from_input=off  hdl_port=on  timing_constraint=None  locs_specified=off  LOCs={}  UseAsDAC=off  DACChannel='1'  block_type=gatewayout
  I_32_30_5 : xbsIndex_r4/Constant  const=0  gui_display_data_type=Fixed-point  arith_type=Signed (2's comp)  n_bits=32  bin_pt=30  preci_type=Single  exp_width=8  frac_width=24  explicit_period=on  period=1  equ=P=C  opselect=C  inp2=PCIN>>17  opr=+  inp1=P  carry=CIN  dbl_ovrd=off  block_type=constant
  Logical : xbsIndex_r4/Logical  logical_function=AND  inputs=2  en=off  latency=0  precision=Full  arith_type=Unsigned  n_bits=16  bin_pt=0  align_bp=on  dbl_ovrd=off  block_type=logical
  Mux{,1..3} (4 alike) : xbsIndex_r4/Mux  inputs=2  en=off  latency=0  precision=Full  arith_type=Unsigned  n_bits=16  bin_pt=14  quantization=Truncate  overflow=Wrap  dbl_ovrd=off  block_type=mux
  PhaseAccum1 : xbsIndex_r4/Single Port RAM  depth=256  initVector=zeros(1,256)  distributed_mem=Block RAM  write_mode=Read After Write  rst=off  init_reg=0  en=off  latency=1  dbl_ovrd=off  optimize=Area  use_rpm=on  block_type=spram
  PhaseIncrement1 : xbsIndex_r4/Single Port RAM  depth=256  initVector=zeros(1,256)  distributed_mem=Block RAM  write_mode=Read After Write  rst=off  init_reg=0  en=off  latency=1  dbl_ovrd=off  optimize=Area  use_rpm=on  block_type=spram
  Relational : xbsIndex_r4/Relational  mode=a!=b  en=off  latency=0  dbl_ovrd=off  block_type=relational
  bit0_ : xbsIndex_r4/Slice  nbits=1  boolean_output=on  mode=Lower Bit Location + Width  bit1=0  base1=MSB of Input  bit0=0  base0=LSB of Input  dbl_ovrd=off  block_type=slice
  bit1_ : xbsIndex_r4/Slice  nbits=1  boolean_output=on  mode=Lower Bit Location + Width  bit1=0  base1=MSB of Input  bit0=1  base0=LSB of Input  dbl_ovrd=off  block_type=slice
  bit7_0_ : xbsIndex_r4/Slice  nbits=8  boolean_output=off  mode=Lower Bit Location + Width  bit1=0  base1=MSB of Input  bit0=0  base0=LSB of Input  dbl_ovrd=off  block_type=slice
  bits_7_0_ : xbsIndex_r4/Slice  nbits=8  boolean_output=off  mode=Lower Bit Location + Width  bit1=0  base1=MSB of Input  bit0=0  base0=LSB of Input  dbl_ovrd=off  block_type=slice
  c2polar_ : Subsystem
  i16_15_ : xbsIndex_r4/Convert  gui_display_data_type=Fixed-point  arith_type="Signed  (2's comp)"  n_bits=16  bin_pt=15  float_type=Single  exp_bits=8  fraction_bits=24  quantization=Truncate  overflow=Wrap  en=off  latency=0  dbl_ovrd=off  pipeline=off  block_type=convert
  i16_15_2 : xbsIndex_r4/Reinterpret  force_arith_type=on  arith_type="Signed  (2's comp)"  force_bin_pt=on  bin_pt=15  block_type=reinterpret
  i18_15_ : xbsIndex_r4/Convert  gui_display_data_type=Fixed-point  arith_type="Signed  (2's comp)"  n_bits=18  bin_pt=15  float_type=Single  exp_bits=8  fraction_bits=24  quantization=Truncate  overflow=Wrap  en=off  latency=0  dbl_ovrd=off  pipeline=off  block_type=convert
  i32_30 : xbsIndex_r4/Reinterpret  force_arith_type=on  arith_type="Signed  (2's comp)"  force_bin_pt=on  bin_pt=30  block_type=reinterpret
  i32_30_ : xbsIndex_r4/Assert  assert_type=on  type_source=Explicitly  gui_display_data_type=Fixed-point  arith_type="Signed  (2's comp)"  n_bits=32  bin_pt=30  preci_type=Single  exp_width=8  frac_width=24  assert_rate=off  rate_source=Explicitly  period=1  output_port=on  block_type=assert
  i32_30_1 : xbsIndex_r4/Assert  assert_type=on  type_source=Explicitly  gui_display_data_type=Fixed-point  arith_type="Signed  (2's comp)"  n_bits=32  bin_pt=30  preci_type=Single  exp_width=8  frac_width=24  assert_rate=off  rate_source=Explicitly  period=1  output_port=on  block_type=assert
  lsb16_ : xbsIndex_r4/Slice  nbits=16  boolean_output=off  mode=Lower Bit Location + Width  bit1=0  base1=MSB of Input  bit0=0  base0=LSB of Input  dbl_ovrd=off  block_type=slice
  phaseCorrScope : Scope  NumInputPorts=8
      settings: YMin=-5~-5~-5~-5~-5~-5~-5~-5  YMax=5~5~5~5~5~5~5~5  SaveName=fsmdata1
  phaseIncAddr : Subsystem  Tag=xps:sw_reg  AncestorBlock=xps_library/software register  mask{numios=1, io_dir=From Processor, io_delay=0, sample_period=1, name1=reg, bitwidth1=32, arith_type1=Unsigned, bin_pt1=0}
      mask prompts: numios "Num I/Os"; io_dir "I/O direction"; io_delay "I/O delay"; sample_period "Sample period"; name1 "Name"; bitwidth1 "Bitwidth"; arith_type1 "Type"; bin_pt1 "Binary pt"
      mask init:
      | swreg_init(gcb);
      mask Callback numios: t = timer('StartDelay', 0.1); t.TimerFcn = {@swreg_cb, gcb}; start(t);
      mask TypeOptions io_dir: To Processor | From Processor
      mask Callback io_dir:
      | a = get_param(gcb, 'MaskEnables');
      | if strcmp(get_param(gcb, 'io_dir'), 'To Processor'),
      | a(4) = {'off'};
      | else
      | a(4) = {'on'};
      | end
      | set_param(gcb, 'MaskEnables', a);
      mask TypeOptions arith_type1: Unsigned | Signed  (2's comp) | Boolean
      mask Callback arith_type1:
      | a = get_param(gcb, 'MaskEnables');
      | if strcmp(get_param(gcb, 'arith_type1'), 'Boolean'),
      | set_param(gcb, 'bitwidth1', '1');
      | set_param(gcb, 'bin_pt1', '0');
      | a(6) = {'off'};
      | a(8) = {'off'};
      | else
      | a(6) = {'on'};
      | a(8) = {'on'};
      | end
      | set_param(gcb, 'MaskEnables', a);
  phaseIncProgWe : Subsystem  Tag=xps:sw_reg  AncestorBlock=xps_library/software register  mask{numios=1, io_dir=From Processor, io_delay=0, sample_period=1, name1=reg, bitwidth1=32, arith_type1=Unsigned, bin_pt1=0}
      mask prompts: numios "Num I/Os"; io_dir "I/O direction"; io_delay "I/O delay"; sample_period "Sample period"; name1 "Name"; bitwidth1 "Bitwidth"; arith_type1 "Type"; bin_pt1 "Binary pt"
      mask init:
      | swreg_init(gcb);
      mask Callback numios: t = timer('StartDelay', 0.1); t.TimerFcn = {@swreg_cb, gcb}; start(t);
      mask TypeOptions io_dir: To Processor | From Processor
      mask Callback io_dir:
      | a = get_param(gcb, 'MaskEnables');
      | if strcmp(get_param(gcb, 'io_dir'), 'To Processor'),
      | a(4) = {'off'};
      | else
      | a(4) = {'on'};
      | end
      | set_param(gcb, 'MaskEnables', a);
      mask TypeOptions arith_type1: Unsigned | Signed  (2's comp) | Boolean
      mask Callback arith_type1:
      | a = get_param(gcb, 'MaskEnables');
      | if strcmp(get_param(gcb, 'arith_type1'), 'Boolean'),
      | set_param(gcb, 'bitwidth1', '1');
      | set_param(gcb, 'bin_pt1', '0');
      | a(6) = {'off'};
      | a(8) = {'off'};
      | else
      | a(6) = {'on'};
      | a(8) = {'on'};
      | end
      | set_param(gcb, 'MaskEnables', a);
  phaseIncVal : Subsystem  Tag=xps:sw_reg  AncestorBlock=xps_library/software register  mask{numios=1, io_dir=From Processor, io_delay=0, sample_period=1, name1=reg, bitwidth1=32, arith_type1=Unsigned, bin_pt1=0}
      mask prompts: numios "Num I/Os"; io_dir "I/O direction"; io_delay "I/O delay"; sample_period "Sample period"; name1 "Name"; bitwidth1 "Bitwidth"; arith_type1 "Type"; bin_pt1 "Binary pt"
      mask init:
      | swreg_init(gcb);
      mask Callback numios: t = timer('StartDelay', 0.1); t.TimerFcn = {@swreg_cb, gcb}; start(t);
      mask TypeOptions io_dir: To Processor | From Processor
      mask Callback io_dir:
      | a = get_param(gcb, 'MaskEnables');
      | if strcmp(get_param(gcb, 'io_dir'), 'To Processor'),
      | a(4) = {'off'};
      | else
      | a(4) = {'on'};
      | end
      | set_param(gcb, 'MaskEnables', a);
      mask TypeOptions arith_type1: Unsigned | Signed  (2's comp) | Boolean
      mask Callback arith_type1:
      | a = get_param(gcb, 'MaskEnables');
      | if strcmp(get_param(gcb, 'arith_type1'), 'Boolean'),
      | set_param(gcb, 'bitwidth1', '1');
      | set_param(gcb, 'bin_pt1', '0');
      | a(6) = {'off'};
      | a(8) = {'off'};
      | else
      | a(6) = {'on'};
      | a(8) = {'on'};
      | end
      | set_param(gcb, 'MaskEnables', a);
  ri_to_c : casper_library_misc/ri_to_c
  ui8_ : xbsIndex_r4/Convert  gui_display_data_type=Fixed-point  arith_type=Unsigned  n_bits=8  bin_pt=0  float_type=Single  exp_bits=8  fraction_bits=24  quantization=Truncate  overflow=Wrap  en=off  latency=0  dbl_ovrd=off  pipeline=off  block_type=convert
  dvld_out : Outport
  cmplx_dout : Outport  Port=2
  chanout : Outport  Port=3
  wires:
  PhaseIncrement1/1 -> Gateway Out/1, i32_30_1/1
  Delay3/1 -> c2polar_/1(c)
  cmplx_din/1 -> Delay3/1
  chan/1 -> Delay/1, ui8_/1
  c2polar_/2(phase) -> lsb16_/1
  AddSub2/1 -> i32_30_/1, i16_15_/1
  dvld_in/1 -> Gateway Out6/1, Logical/1, Delay2/1
  i32_30_/1 -> Mux3/2
  i32_30_1/1 -> AddSub2/1
  ri_to_c/1 -> cmplx_dout/1
  ui8_/1 -> Mux/2, Mux1/2
  Delay1/1 -> ri_to_c/1
  AddSub1/1 -> i18_15_/1
  i16_15_/1 -> Gateway Out1/1, AddSub1/2
  lsb16_/1 -> i16_15_2/1
  i18_15_/1 -> Gateway Out4/1, ri_to_c/2
  en/1 -> [enable], Gateway Out5/1, Logical/2
  Logical/1 -> Mux2/2
  [enable] -> Delay3/2, Delay2/2
  [enable] -> AddSub1/3, Delay1/2
  Delay/1 -> chanout/1
  [enable] -> Delay/2
  i32_30/1 -> PhaseIncrement1/2
  phaseIncVal/1(in_reg) -> i32_30/1
  phaseIncProgWe/1(in_reg) -> bit1_/1, bit0_/1
  bit0_/1 -> PhaseIncrement1/3
  bit1_/1 -> Mux/1
  phaseIncAddr/1(in_reg) -> bit7_0_/1
  bit7_0_/1 -> Mux/3
  From Workspace/1 -> phaseIncVal/1(sim_reg)
  From Workspace1/1 -> phaseIncAddr/1(sim_reg)
  From Workspace2/1 -> phaseIncProgWe/1(sim_reg)
  Mux/1 -> PhaseIncrement1/1
  Mux2/1 -> PhaseAccum1/3
  Mux3/1 -> PhaseAccum1/2
  PhaseAccum1/1 -> AddSub2/2
  I_32_30_5/1 -> Mux3/3
  Constant/1 -> Relational/1
  Counter/1 -> bits_7_0_/1, Relational/2
  clrPhase/1 -> Counter/1
  Relational/1 -> Counter/2, Mux2/1, Mux3/1, Mux1/1, Mux2/3
  bits_7_0_/1 -> Mux1/3
  i16_15_2/1 -> Gateway Out3/1, AddSub1/1
  Gateway Out/1 -> phaseCorrScope/1
  Gateway Out1/1 -> phaseCorrScope/2
  Gateway Out2/1 -> phaseCorrScope/3
  Gateway Out3/1 -> phaseCorrScope/4
  Gateway Out4/1 -> phaseCorrScope/5
  Gateway Out5/1 -> phaseCorrScope/6
  Gateway Out6/1 -> phaseCorrScope/7
  Gateway Out7/1 -> phaseCorrScope/8
  c2polar_/1(power) -> Gateway Out2/1, Delay1/1
  Mux1/1 -> PhaseAccum1/1
  Delay2/1 -> Gateway Out7/1, dvld_out/1
